simulink model "LaneFollowingTestBenchExample"  (R2020a)
settings: Solver=VariableStepAuto  StartTime=0.0  StopTime=simStopTime  RelTol=1e-3
PostLoadFcn:
  | helperLFSetUp
values from neighbouring files (symbols this model uses):
  lr = 1.6    [helperLFSetUp.m]
  m = 1575    [helperLFSetUp.m]
  tau = 0.5    [helperLFSetUp.m]
  Ts = 0.1    [helperLFSetUp.m]
  v_set = egoCar.v0    [helperLFSetUp.m]
undefined symbols (not defined in the file or in its folder): driving
libraries: drivingscenarioandsensors x10, drivinglib x1, autolibshared x1
(part 1 of 3)
CloseFcn:
  | helperLFCleanUp
settings Model: Creator=The MathWorks, Inc.  LastModifiedBy=NAGARJUN
settings DataIOCC: ReturnWorkspaceOutputs=off
settings DebuggingCC: ParameterPrecisionLossMsg=none  PregeneratedLibrarySubsystemCodeDiagnostic=none  ArithmeticOperatorsInVariantConditions=warning
settings HardwareCC: ProdLongLongMode=on
settings SFSimCC: SimUseLocalCustomCode=off
settings RTWCC: GenerateReport=on  RTWUseLocalCustomCode=off  LaunchReport=on
settings ConfigComp: CovScope=ReferencedModels  CovIncludeTopModel=off  CovHtmlReporting=on

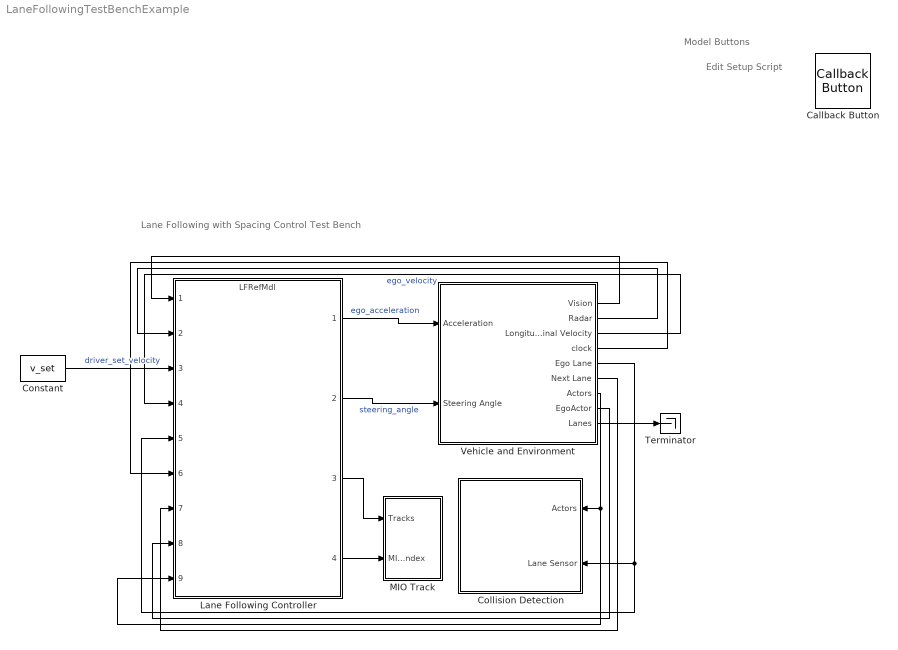
== system LaneFollowingTestBenchExample ==
  note: Edit Setup Script
  note: Lane Following with Spacing Control
      | Test Bench
  note: Model Buttons
  Callback Button : CallbackButton  ButtonText=?
      settings: ClickFcn=|
      | exampleName = 'lane-following-control-with-sensor-fusion-and-lane-detection.html';
      | if license('test','automated_driving_toolbox') && ~isempty(ver('driving'))
      |    web(fullfile(docroot,'driving','examples', exampleName));
      | elseif license('test','MPC_Toolbox') && ~isempty(ver('mpc'))
      |     web(fullfile(docroot,'mpc','ug', exampleName));
      | else
      |     web(fullfile('https://www.mathworks.com/help','driving','examples',exampleName));
      | end
  Collision Detection : Subsystem
  Constant : Constant  Value=v_set  SampleTime=Ts
  Lane Following Controller : ModelReference  ModelNameDialog=LFRefMdl  SimulationMode=Normal  CodeInterface=Top model  ModelReferenceVersion=1.766
  MIO Track : Subsystem
  Terminator : Terminator
  Vehicle and Environment : Subsystem
  wires:
  Lane Following Controller/1 -> Vehicle and Environment/1(Acceleration)  "ego_acceleration"
  Lane Following Controller/2 -> Vehicle and Environment/2(Steering Angle)  "steering_angle"
  Constant/1 -> Lane Following Controller/3  "driver_set_velocity"
  Vehicle and Environment/3(Longitudinal Velocity) -> Lane Following Controller/4  "ego_velocity"
  Vehicle and Environment/5(Ego Lane) -> Lane Following Controller/5, Collision Detection/2(Lane Sensor)
  Vehicle and Environment/2(Radar) -> Lane Following Controller/2
  Vehicle and Environment/1(Vision) -> Lane Following Controller/1
  Lane Following Controller/3 -> MIO Track/1(Tracks)
  Lane Following Controller/4 -> MIO Track/2(MIO Index)
  Vehicle and Environment/7(Actors) -> Lane Following Controller/9, Collision Detection/1(Actors)
  Vehicle and Environment/4(clock) -> Lane Following Controller/6
  Vehicle and Environment/6(Next Lane) -> Lane Following Controller/7
  Vehicle and Environment/8(EgoActor) -> Lane Following Controller/8
  Vehicle and Environment/9(Lanes) -> Terminator/1

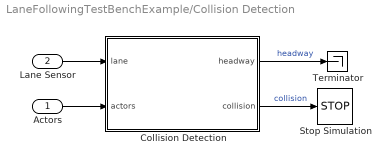
== system LaneFollowingTestBenchExample/Collision Detection ==
  Actors : Inport
  Lane Sensor : Inport  Port=2
  Collision Detection : MATLAB Function  TreatAsAtomicUnit=on
  Stop Simulation : Stop
  Terminator : Terminator
  wires:
  Collision Detection/2(collision) -> Stop Simulation/1  "collision"
  Actors/1 -> Collision Detection/2(actors)
  Lane Sensor/1 -> Collision Detection/1(lane)
  Collision Detection/1(headway) -> Terminator/1  "headway"

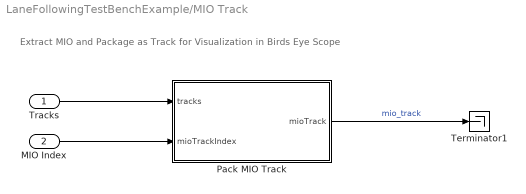
== system LaneFollowingTestBenchExample/MIO Track ==
  note: Extract MIO and Package as Track for Visualization in Birds Eye Scope
  Tracks : Inport
  MIO Index : Inport  Port=2
  Pack MIO Track : MATLAB Function  TreatAsAtomicUnit=on
  Terminator1 : Terminator
  wires:
  Tracks/1 -> Pack MIO Track/1(tracks)
  Pack MIO Track/1(mioTrack) -> Terminator1/1  "mio_track"
  MIO Index/1 -> Pack MIO Track/2(mioTrackIndex)

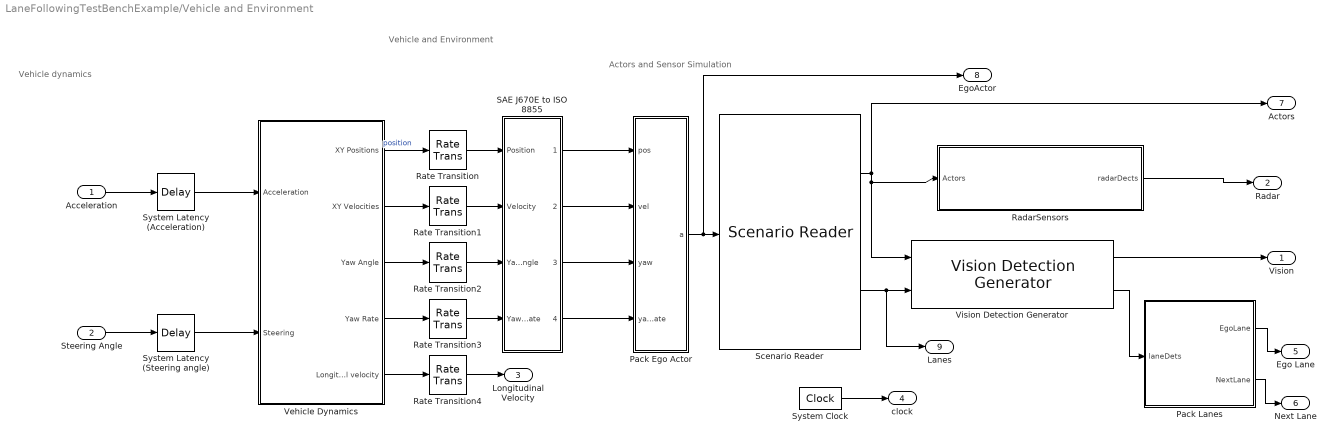
== system LaneFollowingTestBenchExample/Vehicle and Environment ==
  note: Vehicle dynamics
  note: Actors and Sensor Simulation
  note: Vehicle and Environment
  Acceleration : Inport  Unit=m/s^2
  Steering Angle : Inport  Port=2  Unit=rad
  Pack Ego Actor : MATLAB Function  TreatAsAtomicUnit=on
  Pack Lanes : MATLAB Function  TreatAsAtomicUnit=on
  RadarSensors : Subsystem
  Rate Transition{,1..4} (5 alike) : RateTransition  OutPortSampleTime=Ts
  SAE J670E to ISO 8855 : Subsystem
  Scenario Reader : drivingscenarioandsensors/Scenario Reader  ScenarioSource=From file  ScenarioFileName=mySin_LF_03__DbCurve.mat  ScenarioVariableName=scenario  OutputCoordinateSystem=Vehicle coordinates  EgoVehicleSource=Input port  OrientVehiclesOnRoad=off  EgoVehicleActorID=1  OutputEgoVehiclePose=off  SampleTime=0.1  LaneBoundaryOutput=Ego vehicle lane boundaries  LaneBoundaryDistance=0:0.5:60  LaneBoundaryLocation=Inner edge of lane markings  BusNameSource=Auto  BusName=BusActors  BusName2Source=Auto  BusName2=BusLaneBoundaries  BusName3Source=Auto  BusName3=BusEgoActor  ShowCoordinateLabels=on  SimulateUsing=Interpreted execution
  System Clock : DigitalClock  SampleTime=Ts
  System Latency (Acceleration) : TransportDelay  DelayTime=Ts
  System Latency (Steering angle) : TransportDelay  DelayTime=Ts
  Vehicle Dynamics : Subsystem  VariantControl=Variant2
  Vision Detection Generator : drivingscenarioandsensors/Vision Detection Generator  SensorIndex=1  DetectorOutput=Lanes and objects  UpdateInterval=0.1  LaneUpdateInterval=0.1  SensorLocation=[ 3.22, 0 ]  Height=1.1  Yaw=0  Pitch=1  Roll=0  BusNameSource=Property  BusName=BusVision  BusName2Source=Property  BusName2=BusLanes  MaxNumDetectionsSource=Property  MaxNumDetections=20  MaxNumLanesSource=Property  MaxNumLanes=2  DetectionCoordinates=Ego Cartesian  SimulateUsing=Interpreted execution  MaxRange=150  BoundingBoxAccuracy=5  ProcessNoiseIntensity=5  MaxSpeed=50  MaxAllowedOcclusion=0.5  MinObjectImageSize=[ 10, 10 ]  DetectionProbability=0.9  FalsePositivesPerImage=0.1  MinLaneImageSize=[ 20, 3 ]  LaneBoundaryAccuracy=3  HasNoise=on  InitialSeedSource=Repeatable  InitialSeed=0  UsedSeed=driving.internal.SimulinkUtilities.seedManager(gcb)  ActorProfilesSource=MATLAB expression  ActorProfilesParameters=driving.internal.ActorProfilesParameters  ActorProfilesExpression=actor_Profiles  Intrinsics=driving.internal.cameraIntrinsics('FocalLength',[ 800,800 ])
  Vision : Outport  VectorParamsAs1DForOutWhenUnconnected=off
  Radar : Outport  Port=2  VectorParamsAs1DForOutWhenUnconnected=off
  Longitudinal Velocity : Outport  Port=3  VectorParamsAs1DForOutWhenUnconnected=off
  clock : Outport  Port=4
  Ego Lane : Outport  Port=5  VectorParamsAs1DForOutWhenUnconnected=off
  Next Lane : Outport  Port=6  VectorParamsAs1DForOutWhenUnconnected=off
  Actors : Outport  Port=7  VectorParamsAs1DForOutWhenUnconnected=off
  EgoActor : Outport  Port=8
  Lanes : Outport  Port=9
  wires:
  Scenario Reader/1 -> RadarSensors/1(Actors), Vision Detection Generator/1, Actors/1
  Vehicle Dynamics/2(XY Velocities) -> Rate Transition1/1
  Vehicle Dynamics/3(Yaw Angle) -> Rate Transition2/1
  Vehicle Dynamics/4(Yaw Rate) -> Rate Transition3/1
  Vehicle Dynamics/1(XY Positions) -> Rate Transition/1  "position"
  Rate Transition4/1 -> Longitudinal Velocity/1
  Vehicle Dynamics/5(Longitudinal velocity) -> Rate Transition4/1
  Scenario Reader/2 -> Lanes/1, Vision Detection Generator/2
  Vision Detection Generator/1 -> Vision/1
  Acceleration/1 -> System Latency (Acceleration)/1
  Steering Angle/1 -> System Latency (Steering angle)/1
  System Latency (Acceleration)/1 -> Vehicle Dynamics/1(Acceleration)
  System Latency (Steering angle)/1 -> Vehicle Dynamics/2(Steering)
  SAE J670E to ISO 8855/1(1) -> Pack Ego Actor/1(pos)
  SAE J670E to ISO 8855/2(2) -> Pack Ego Actor/2(vel)
  SAE J670E to ISO 8855/3(3) -> Pack Ego Actor/3(yaw)
  SAE J670E to ISO 8855/4(4) -> Pack Ego Actor/4(yawRate)
  Rate Transition3/1 -> SAE J670E to ISO 8855/4(Yaw Rate)
  Rate Transition2/1 -> SAE J670E to ISO 8855/3(Yaw Angle)
  Rate Transition1/1 -> SAE J670E to ISO 8855/2(Velocity)
  Rate Transition/1 -> SAE J670E to ISO 8855/1(Position)
  Vision Detection Generator/2 -> Pack Lanes/1(laneDets)
  Pack Lanes/2(NextLane) -> Next Lane/1
  Pack Lanes/1(EgoLane) -> Ego Lane/1
  System Clock/1 -> clock/1
  RadarSensors/1(radarDects) -> Radar/1
  Pack Ego Actor/1(a) -> EgoActor/1, Scenario Reader/1

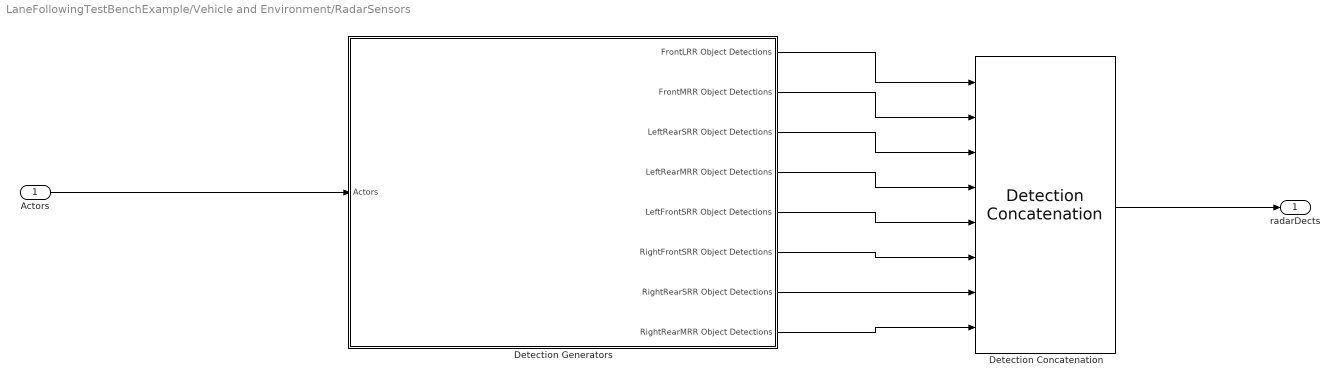
== system LaneFollowingTestBenchExample/Vehicle and Environment/RadarSensors ==
  Actors : Inport
  Detection Concatenation : drivinglib/Detection Concatenation  NumInputs=8  BusNameSource=Auto  BusName=BusDetectionConcatenation  SimulateUsing=Interpreted execution
      settings: SourceProductBaseCode=DR
  Detection Generators : Subsystem
  radarDects : Outport
  wires:
  Detection Generators/7(RightRearSRR Object Detections) -> Detection Concatenation/7
  Detection Generators/1(FrontLRR Object Detections) -> Detection Concatenation/1
  Detection Generators/2(FrontMRR Object Detections) -> Detection Concatenation/2
  Detection Generators/6(RightFrontSRR Object Detections) -> Detection Concatenation/6
  Detection Concatenation/1 -> radarDects/1
  Detection Generators/3(LeftRearSRR Object Detections) -> Detection Concatenation/3
  Detection Generators/4(LeftRearMRR Object Detections) -> Detection Concatenation/4
  Detection Generators/5(LeftFrontSRR Object Detections) -> Detection Concatenation/5
  Detection Generators/8(RightRearMRR Object Detections) -> Detection Concatenation/8
  Actors/1 -> Detection Generators/1(Actors)

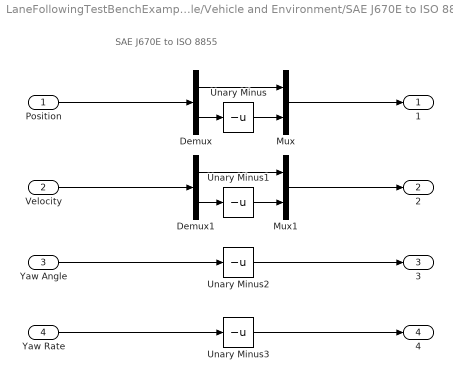
== system LaneFollowingTestBenchExample/Vehicle and Environment/SAE J670E to ISO 8855 ==
  note: SAE J670E to ISO 8855
  Position : Inport  Unit=m
  Velocity : Inport  Port=2  Unit=m/s
  Yaw Angle : Inport  Port=3  Unit=deg
  Yaw Rate : Inport  Port=4  Unit=deg/s
  Demux : Demux  Outputs=2
  Demux1 : Demux  Outputs=2
  Mux : Mux  Inputs=2
  Mux1 : Mux  Inputs=2
  Unary Minus{,1..3} (4 alike) : UnaryMinus
  1 : Outport  VectorParamsAs1DForOutWhenUnconnected=off
  2 : Outport  Port=2  VectorParamsAs1DForOutWhenUnconnected=off
  3 : Outport  Port=3  VectorParamsAs1DForOutWhenUnconnected=off
  4 : Outport  Port=4  VectorParamsAs1DForOutWhenUnconnected=off
  wires:
  Yaw Rate/1 -> Unary Minus3/1
  Yaw Angle/1 -> Unary Minus2/1
  Demux/1 -> Mux/1
  Demux/2 -> Unary Minus/1
  Unary Minus/1 -> Mux/2
  Unary Minus1/1 -> Mux1/2
  Demux1/2 -> Unary Minus1/1
  Demux1/1 -> Mux1/1
  Mux1/1 -> 2/1
  Mux/1 -> 1/1
  Position/1 -> Demux/1
  Velocity/1 -> Demux1/1
  Unary Minus2/1 -> 3/1
  Unary Minus3/1 -> 4/1

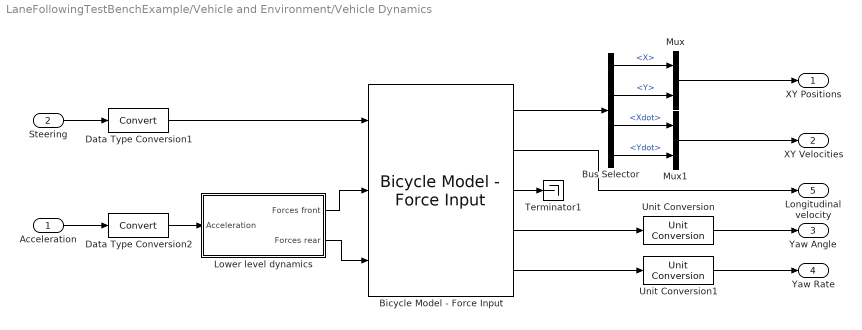
== system LaneFollowingTestBenchExample/Vehicle and Environment/Vehicle Dynamics ==
  Acceleration : Inport  Unit=m/s^2
  Steering : Inport  Port=2  Unit=rad
  Bicycle Model - Force Input : autolibshared/Bicycle Model - Force Input  trackMode=Single (bicycle)  inputMode=External longitudinal forces  frontSteerMode=on  rearSteerMode=off  windMode=off  muMode=off  extFMode=off  extMMode=off  aMode=3  NF=2  NR=2  m=m  a=lf  b=lr  h=0.35  X_o=x0_ego  xdot_o=v0_ego  CalphaMode=off  sigmaMode=on  w=[1.4,1.4]  Cy_f=Cf  Cy_r=Cr  sigma_f=.1  sigma_r=.1  alpha_f_brk=[-.1 .1]  Cy_f_data=[-9e3 9e3]  alpha_r_brk=[-.1 .1]  Cy_r_data=[-9e3 9e3]  Y_o=y0_ego  ydot_o=0  Izz=Iz  psi_o=yaw0_ego  r_o=0  Af=0  Cd=.3  Cl=.1  Cpm=.1  beta_w=[0:0.01:0.3]  Cs=[0:0.03:0.9]  Cym=[0:0.01:0.3]  Pabs=101325  Tair=273  g=9.81  mu=1  xdot_tol=.01  Fznom=5000  Fxtire_sat=1e6  Fytire_sat=1e6  longOff=0  latOff=0  vertOff=0
      settings: SourceProductBaseCode=PW,MT,VE,VP
  Bus Selector : BusSelector  OutputSignals=InertFrm.FrntAxl.Disp.X,InertFrm.FrntAxl.Disp.Y,InertFrm.FrntAxl.Vel.Xdot,InertFrm.FrntAxl.Vel.Ydot
  Data Type Conversion1 : DataTypeConversion
  Data Type Conversion2 : DataTypeConversion
  Lower level dynamics : Subsystem
  Mux : Mux  Inputs=2
  Mux1 : Mux  Inputs=2
  Terminator1 : Terminator
  Unit Conversion : UnitConversion  OutputType=Inherit: Inherit via back propagation
  Unit Conversion1 : UnitConversion  OutputType=Inherit: Inherit via back propagation
  XY Positions : Outport  Unit=m  VectorParamsAs1DForOutWhenUnconnected=off
  XY Velocities : Outport  Port=2  Unit=m/s  VectorParamsAs1DForOutWhenUnconnected=off
  Yaw Angle : Outport  Port=3  Unit=deg  VectorParamsAs1DForOutWhenUnconnected=off
  Yaw Rate : Outport  Port=4  Unit=degree/s  VectorParamsAs1DForOutWhenUnconnected=off
  Longitudinal velocity : Outport  Port=5  VectorParamsAs1DForOutWhenUnconnected=off
  wires:
  Lower level dynamics/2(Forces rear) -> Bicycle Model - Force Input/3
  Lower level dynamics/1(Forces front) -> Bicycle Model - Force Input/2
  Data Type Conversion2/1 -> Lower level dynamics/1(Acceleration)
  Data Type Conversion1/1 -> Bicycle Model - Force Input/1
  Acceleration/1 -> Data Type Conversion2/1
  Steering/1 -> Data Type Conversion1/1
  Bus Selector/1 -> Mux/1  "<X>"
  Unit Conversion/1 -> Yaw Angle/1
  Bicycle Model - Force Input/5 -> Unit Conversion1/1
  Bus Selector/4 -> Mux1/2  "<Ydot>"
  Bicycle Model - Force Input/4 -> Unit Conversion/1
  Bus Selector/2 -> Mux/2  "<Y>"
  Bicycle Model - Force Input/2 -> Longitudinal velocity/1
  Bus Selector/3 -> Mux1/1  "<Xdot>"
  Bicycle Model - Force Input/1 -> Bus Selector/1
  Bicycle Model - Force Input/3 -> Terminator1/1
  Mux/1 -> XY Positions/1
  Mux1/1 -> XY Velocities/1
  Unit Conversion1/1 -> Yaw Rate/1
